simulink library "UpmixerLib"  (R2022b)
settings: Solver=VariableStepAuto  StartTime=0.0  StopTime=10.0  RelTol=1e-3
undefined symbols (not defined in the file or in its folder): carModel, mode, upmixer
libraries: TuneVar x40, MixerLib x31, $bdroot x13, FeaturePath x6, RTC x4
settings Model: Creator=ak1044356  LastModifiedBy=sa1045272
settings SolverCC: AlgebraicLoopSolver=TrustRegion
settings DebuggingCC: UnconnectedInputMsg=warning  UnconnectedOutputMsg=warning  UnconnectedLineMsg=warning  SFMachineParentedDataDiag=warning  ArithmeticOperatorsInVariantConditions=warning
settings ModelReferenceCC: EnableRefExpFcnMdlSchedulingChecks=on
settings SFSimCC: CustomCodeUndefinedFunction=UseInterfaceOnly

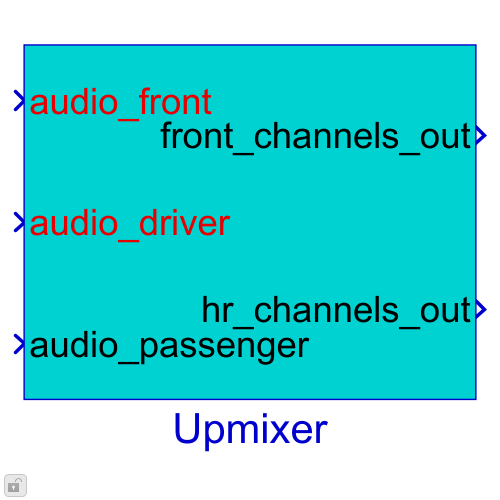
[thumbnail: Simulink's stored preview of the top-level diagram]
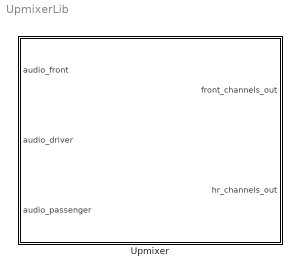
== system UpmixerLib ==
  Upmixer : Subsystem  InitFcn=|
      | upmixer.front_peripheral_channel_count = min(upmixer.front_peripheral_channel_count, 7);
      | upmixer.front_peripheral_channel_count = max(upmixer.front_peripheral_channel_count, 2);
      | upmixer.headrest_count = min(upmixer.headrest_count, 2);
      | upmixer.headrest_count = max(upmixer.headrest_count, 1);

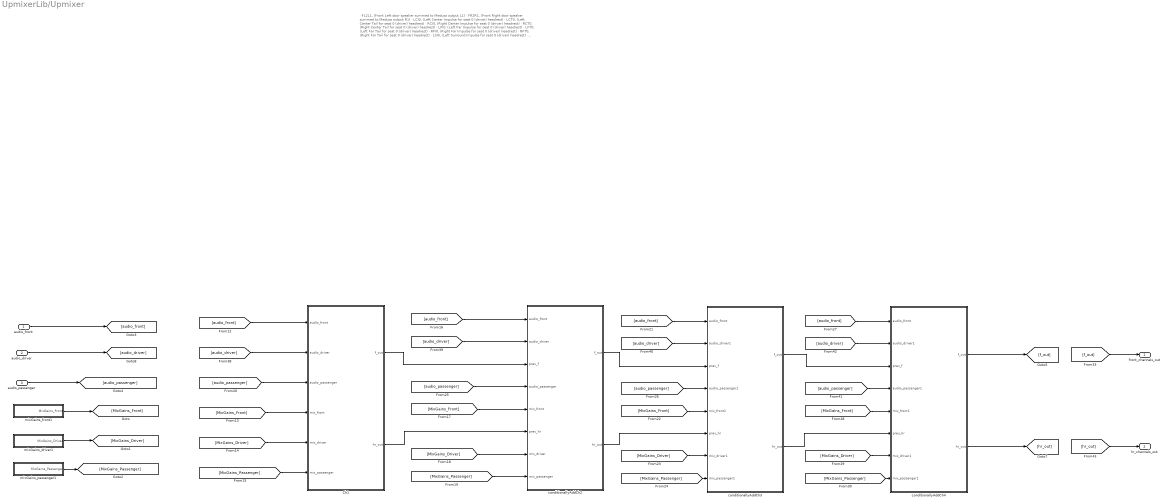
== system UpmixerLib/Upmixer ==
  note: · FL2L1, (Front Left door speaker summed to Medusa output L1)
      | · FR2R1, (Front Right door speaker summed to Medusa output R1)
      | · LCI0, (Left Center Impulse for seat 0 (driver) headrest)
      | · LCT0, (Left Center Tail for seat 0 (driver) headrest)
      | · RCI0, (Right Center Impulse for seat 0 (driver) headrest)
      | · RCT0, (Right Center Tail for seat 0 (driver) headrest)
      | · LFI0, (Left Far Impulse for seat 0 (driver) headrest)
      | · LFT0, (Left Far Tail for seat 0 (driver) headrest)
      | · RFI0, (Right Far Impulse for seat 0 (driver) headrest)
      | · RFT0, (Right Far Tail for seat 0 (driver) headrest)
      | · LSI0, (Left Surround Impulse for seat 0 (driver) headrest)
      | · LST0, (Left Surround Tail for seat 0 (driver) headrest)
      | · RSI0, (Right Surround Impulse for seat 0 (driver) headrest)
      | · RST0 (Right Surround Tail for seat 0 (driver) headrest)
  audio_front : Inport
  audio_driver : Inport  Port=2
  audio_passenger : Inport  Port=3
  Ch1 : Subsystem
  conditionallyAddCh2 : Subsystem
  conditionallyAddCh3 : Subsystem  AncestorBlock=UpmixerLib/Upmixer/conditionallyAddCh2
      settings: LibrarySourceBlock=UpmixerLib/Upmixer/conditionallyAddCh2
  conditionallyAddCh4 : Subsystem  AncestorBlock=UpmixerLib/Upmixer/conditionallyAddCh2
      settings: LibrarySourceBlock=UpmixerLib/Upmixer/conditionallyAddCh2
  mixGains_driver1 : Subsystem
  mixGains_front1 : Subsystem
  mixGains_passenger1 : Subsystem
  front_channels_out : Outport  VectorParamsAs1DForOutWhenUnconnected=off
  hr_channels_out : Outport  Port=2  VectorParamsAs1DForOutWhenUnconnected=off
  wires:
  mixGains_front1/1(MixGains_Front) -> [MixGains_Front]
  mixGains_driver1/1(MixGains_Driver) -> [MixGains_Driver]
  mixGains_passenger1/1(MixGains_Passenger) -> [MixGains_Passenger]
  audio_front/1 -> [audio_front]
  [audio_front] -> conditionallyAddCh2/1(audio_front)
  [MixGains_Front] -> conditionallyAddCh2/5(mix_front)
  [MixGains_Driver] -> conditionallyAddCh2/7(mix_driver)
  [MixGains_Passenger] -> conditionallyAddCh2/8(mix_passenger)
  [f_out] -> front_channels_out/1
  audio_driver/1 -> [audio_driver]
  [audio_driver] -> conditionallyAddCh2/2(audio_driver)
  [audio_front] -> Ch1/1(audio_front)
  [audio_driver] -> Ch1/2(audio_driver)
  [MixGains_Front] -> Ch1/4(mix_front)
  [MixGains_Driver] -> Ch1/5(mix_driver)
  [MixGains_Passenger] -> Ch1/6(mix_passenger)
  conditionallyAddCh4/1(f_out) -> [f_out]
  audio_passenger/1 -> [audio_passenger]
  [audio_passenger] -> Ch1/3(audio_passenger)
  [audio_passenger] -> conditionallyAddCh2/4(audio_passenger)
  Ch1/1(f_out) -> conditionallyAddCh2/3(prev_f)
  Ch1/2(hr_out) -> conditionallyAddCh2/6(prev_hr)
  [MixGains_Front] -> conditionallyAddCh3/5(mix_front1)
  [audio_front] -> conditionallyAddCh3/1(audio_front)
  [MixGains_Passenger] -> conditionallyAddCh3/8(mix_passenger1)
  [audio_driver] -> conditionallyAddCh3/2(audio_driver1)
  [audio_passenger] -> conditionallyAddCh3/4(audio_passenger1)
  [MixGains_Driver] -> conditionallyAddCh3/7(mix_driver1)
  conditionallyAddCh2/2(hr_out) -> conditionallyAddCh3/6(prev_hr)
  conditionallyAddCh2/1(f_out) -> conditionallyAddCh3/3(prev_f)
  conditionallyAddCh3/1(f_out) -> conditionallyAddCh4/3(prev_f)
  conditionallyAddCh3/2(hr_out) -> conditionallyAddCh4/6(prev_hr)
  [audio_front] -> conditionallyAddCh4/1(audio_front)
  [audio_driver] -> conditionallyAddCh4/2(audio_driver1)
  [audio_passenger] -> conditionallyAddCh4/4(audio_passenger1)
  [MixGains_Front] -> conditionallyAddCh4/5(mix_front1)
  [MixGains_Driver] -> conditionallyAddCh4/7(mix_driver1)
  [MixGains_Passenger] -> conditionallyAddCh4/8(mix_passenger1)
  conditionallyAddCh4/2(hr_out) -> [hr_out]
  [hr_out] -> hr_channels_out/1

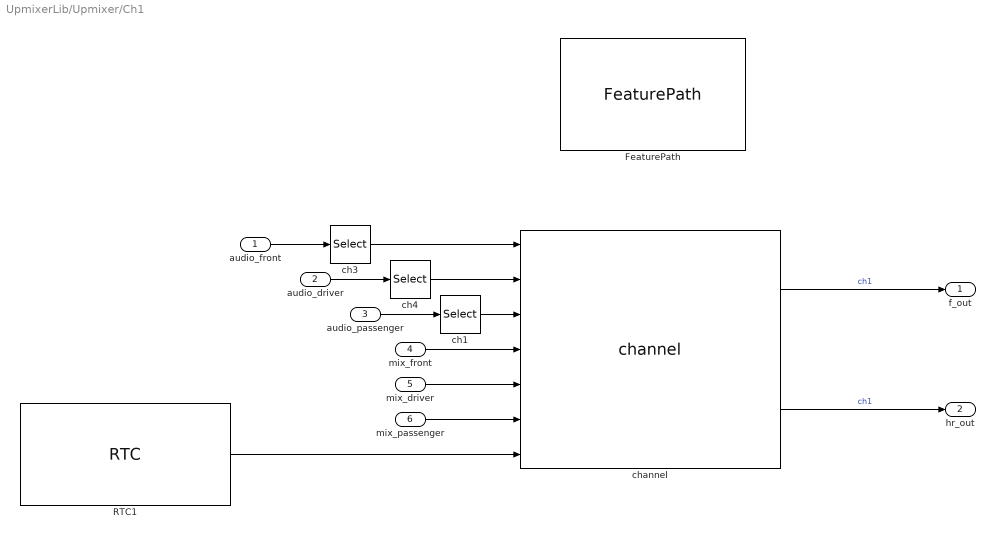
== system UpmixerLib/Upmixer/Ch1 ==
  audio_front : Inport
  audio_driver : Inport  Port=2
  audio_passenger : Inport  Port=3
  mix_front : Inport  Port=4
  mix_driver : Inport  Port=5
  mix_passenger : Inport  Port=6
  FeaturePath : FeaturePath/FeaturePath  FeatureName=Channel1_  IsGroup=off  GroupNumber=-1  DeclarePackages=off  PackageNames=mode,carModel  IsToolGroup=off  TriggerInit=[310 -171 495 -59]
  RTC1 : RTC/RTC  REQ_Priority=RTC_Mask.NormalPriority  RequestAtInit=off  EnableRequest=off  REQElemName1=loc  REQElemType1=single  REQElemWidth1=2  REQElemInitial1=upmixer.loc_init  REQElemType2=uint32  REQElemWidth2=1  REQElemInitial2=[]  REQElemType3=uint32  REQElemWidth3=1  REQElemInitial3=[]  REQElemType4=uint32  REQElemWidth4=1  REQElemInitial4=[]  REQElemType5=uint32  REQElemWidth5=1  REQElemInitial5=[]  REQElemType6=uint32  REQElemWidth6=1  REQElemInitial6=[]  REQElemType7=uint32  REQElemWidth7=1  REQElemInitial7=[]  REQElemType8=uint32  REQElemWidth8=1  REQElemInitial8=[]  REQElemType9=uint32  REQElemWidth9=1  REQElemInitial9=[]  REQElemType10=uint32  REQElemWidth10=1  REQElemInitial10=[]  EnableResponse=on  EnableRSP_StatusIn=off  RSPElemType1=single  RSPElemWidth1=1  RSPElemType2=uint32  RSPElemWidth2=1  RSPElemType3=uint32  RSPElemWidth3=1  RSPElemType4=uint32  RSPElemWidth4=1  RSPElemType5=uint32  RSPElemWidth5=1  RSPElemType6=uint32  RSPElemWidth6=1  RSPElemType7=uint32  RSPElemWidth7=1  RSPElemType8=uint32  RSPElemWidth8=1  RSPElemType9=uint32  RSPElemWidth9=1  RSPElemType10=uint32  RSPElemWidth10=1  EnableNotification=off  EnableNTF_PrepTrig=off  NTFElemType1=uint32  NTFElemWidth1=1  NTFElemType2=uint32  NTFElemWidth2=1  NTFElemType3=uint32  NTFElemWidth3=1  NTFElemType4=uint32  NTFElemWidth4=1  NTFElemType5=uint32  NTFElemWidth5=1  NTFElemType6=uint32  NTFElemWidth6=1  NTFElemType7=uint32  NTFElemWidth7=1  NTFElemType8=uint32  NTFElemWidth8=1  NTFElemType9=uint32  NTFElemWidth9=1  NTFElemType10=uint32  NTFElemWidth10=1  MaskMessageName=Location
  ch1 : Selector  NumberOfDimensions=2  InputPortWidth=3  IndexOptions=Select all,Index vector (dialog)  Indices=4,min(1, upmixer.ann_sysin_channel_count)  OutputSizes=1,1
  ch3 : Selector  NumberOfDimensions=2  InputPortWidth=3  IndexOptions=Select all,Index vector (dialog)  Indices=4,min(1, upmixer.ann_sysin_channel_count)  OutputSizes=1,1
  ch4 : Selector  NumberOfDimensions=2  InputPortWidth=3  IndexOptions=Select all,Index vector (dialog)  Indices=4,min(1, upmixer.ann_sysin_channel_count)  OutputSizes=1,1
  channel : $bdroot/Upmixer/conditionallyAddCh2/If Action Subsystem1/channel  SystemSampleTime=-1  VariantActivationTime=update diagram  Latency=0  AutoFrameSizeCalculation=off
  f_out : Outport  VectorParamsAs1DForOutWhenUnconnected=off
  hr_out : Outport  Port=2  VectorParamsAs1DForOutWhenUnconnected=off
  wires:
  mix_front/1 -> channel/4
  audio_front/1 -> ch3/1
  mix_driver/1 -> channel/5
  mix_passenger/1 -> channel/6
  channel/1 -> f_out/1  "ch1"
  audio_driver/1 -> ch4/1
  RTC1/1 -> channel/7
  audio_passenger/1 -> ch1/1
  ch1/1 -> channel/3
  ch4/1 -> channel/2
  ch3/1 -> channel/1
  channel/2 -> hr_out/1  "ch1"

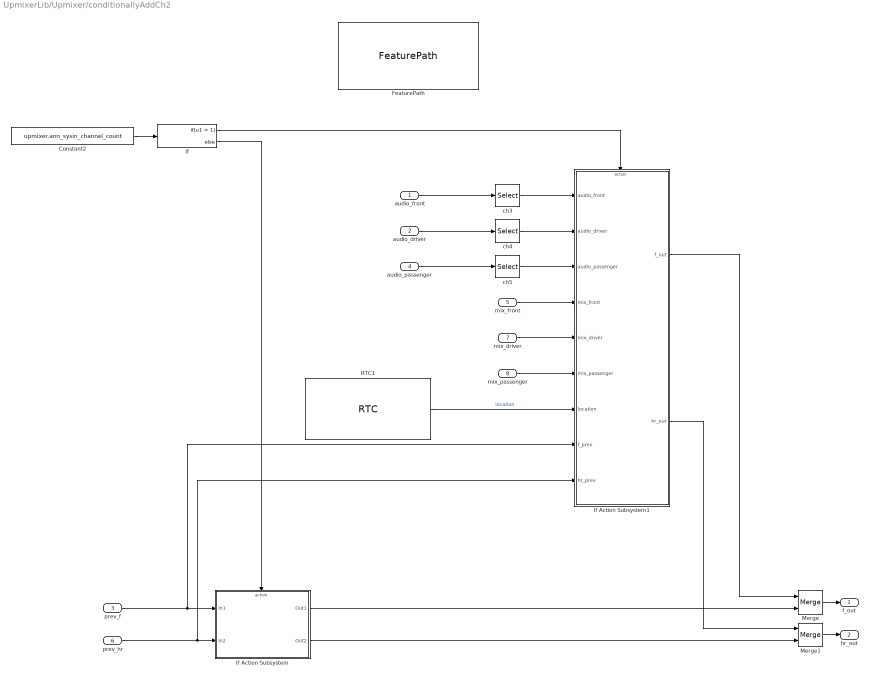
== system UpmixerLib/Upmixer/conditionallyAddCh2 ==
  audio_front : Inport
  audio_driver : Inport  Port=2
  prev_f : Inport  Port=3
  audio_passenger : Inport  Port=4
  mix_front : Inport  Port=5
  prev_hr : Inport  Port=6
  mix_driver : Inport  Port=7
  mix_passenger : Inport  Port=8
  Constant2 : Constant  Value=upmixer.ann_sysin_channel_count
  FeaturePath : FeaturePath/FeaturePath  FeatureName=Channel2_  IsGroup=off  GroupNumber=-1  DeclarePackages=off  PackageNames=mode,carModel  IsToolGroup=off  TriggerInit=[515 -436 750 -324]
  If : If  IfExpression=u1 > 1
  If Action Subsystem : Subsystem  TreatAsAtomicUnit=on
  If Action Subsystem1 : Subsystem  TreatAsAtomicUnit=on
  Merge : Merge
  Merge1 : Merge
  RTC1 : RTC/RTC  REQ_Priority=RTC_Mask.NormalPriority  RequestAtInit=off  EnableRequest=off  REQElemName1=loc  REQElemType1=single  REQElemWidth1=2  REQElemInitial1=upmixer.loc_init  REQElemType2=uint32  REQElemWidth2=1  REQElemInitial2=[]  REQElemType3=uint32  REQElemWidth3=1  REQElemInitial3=[]  REQElemType4=uint32  REQElemWidth4=1  REQElemInitial4=[]  REQElemType5=uint32  REQElemWidth5=1  REQElemInitial5=[]  REQElemType6=uint32  REQElemWidth6=1  REQElemInitial6=[]  REQElemType7=uint32  REQElemWidth7=1  REQElemInitial7=[]  REQElemType8=uint32  REQElemWidth8=1  REQElemInitial8=[]  REQElemType9=uint32  REQElemWidth9=1  REQElemInitial9=[]  REQElemType10=uint32  REQElemWidth10=1  REQElemInitial10=[]  EnableResponse=on  EnableRSP_StatusIn=off  RSPElemType1=single  RSPElemWidth1=1  RSPElemType2=uint32  RSPElemWidth2=1  RSPElemType3=uint32  RSPElemWidth3=1  RSPElemType4=uint32  RSPElemWidth4=1  RSPElemType5=uint32  RSPElemWidth5=1  RSPElemType6=uint32  RSPElemWidth6=1  RSPElemType7=uint32  RSPElemWidth7=1  RSPElemType8=uint32  RSPElemWidth8=1  RSPElemType9=uint32  RSPElemWidth9=1  RSPElemType10=uint32  RSPElemWidth10=1  EnableNotification=off  EnableNTF_PrepTrig=off  NTFElemType1=uint32  NTFElemWidth1=1  NTFElemType2=uint32  NTFElemWidth2=1  NTFElemType3=uint32  NTFElemWidth3=1  NTFElemType4=uint32  NTFElemWidth4=1  NTFElemType5=uint32  NTFElemWidth5=1  NTFElemType6=uint32  NTFElemWidth6=1  NTFElemType7=uint32  NTFElemWidth7=1  NTFElemType8=uint32  NTFElemWidth8=1  NTFElemType9=uint32  NTFElemWidth9=1  NTFElemType10=uint32  NTFElemWidth10=1  MaskMessageName=Location
  ch3 : Selector  NumberOfDimensions=2  InputPortWidth=3  IndexOptions=Select all,Index vector (dialog)  Indices=4,min(2, upmixer.ann_sysin_channel_count)  OutputSizes=1,1
  ch4 : Selector  NumberOfDimensions=2  InputPortWidth=3  IndexOptions=Select all,Index vector (dialog)  Indices=4,min(2, upmixer.ann_sysin_channel_count)  OutputSizes=1,1
  ch5 : Selector  NumberOfDimensions=2  InputPortWidth=3  IndexOptions=Select all,Index vector (dialog)  Indices=4,min(2, upmixer.ann_sysin_channel_count)  OutputSizes=1,1
  f_out : Outport  VectorParamsAs1DForOutWhenUnconnected=off
  hr_out : Outport  Port=2  VectorParamsAs1DForOutWhenUnconnected=off
  wires:
  Constant2/1 -> If/1
  If/2 -> If Action Subsystem/Action
  prev_f/1 -> If Action Subsystem1/8(f_prev), If Action Subsystem/1(In1)
  If/1 -> If Action Subsystem1/Action
  audio_front/1 -> ch3/1
  If Action Subsystem/1(Out1) -> Merge/2
  If Action Subsystem1/1(f_out) -> Merge/1
  Merge/1 -> f_out/1
  mix_front/1 -> If Action Subsystem1/4(mix_front)
  mix_driver/1 -> If Action Subsystem1/5(mix_driver)
  mix_passenger/1 -> If Action Subsystem1/6(mix_passenger)
  RTC1/1 -> If Action Subsystem1/7(location)  "location"
  ch3/1 -> If Action Subsystem1/1(audio_front)
  audio_driver/1 -> ch4/1
  ch4/1 -> If Action Subsystem1/2(audio_driver)
  audio_passenger/1 -> ch5/1
  ch5/1 -> If Action Subsystem1/3(audio_passenger)
  prev_hr/1 -> If Action Subsystem1/9(hr_prev), If Action Subsystem/2(In2)
  If Action Subsystem/2(Out2) -> Merge1/2
  If Action Subsystem1/2(hr_out) -> Merge1/1
  Merge1/1 -> hr_out/1

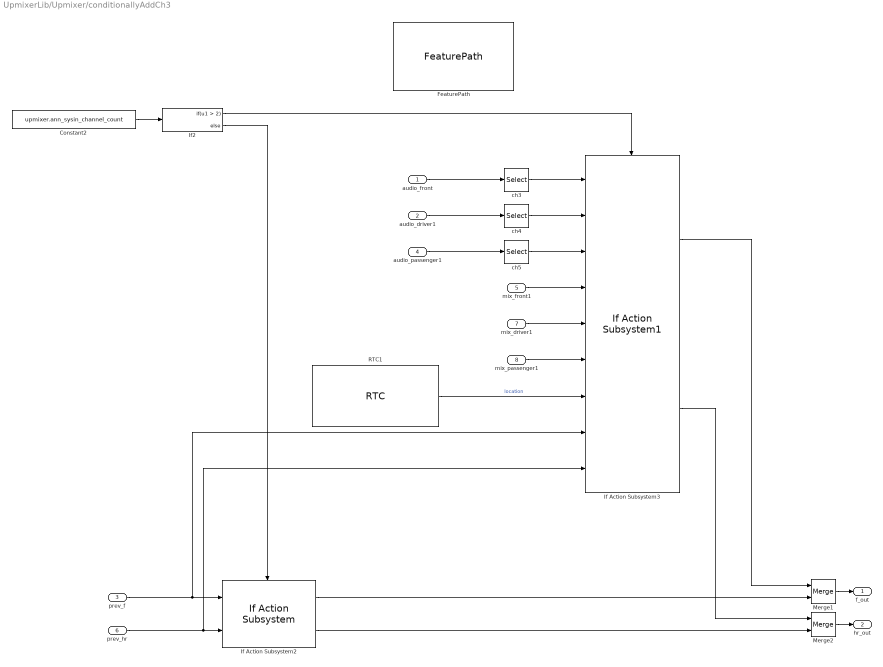
== system UpmixerLib/Upmixer/conditionallyAddCh3 ==
  audio_front : Inport
  audio_driver1 : Inport  Port=2
  prev_f : Inport  Port=3
  audio_passenger1 : Inport  Port=4
  mix_front1 : Inport  Port=5
  prev_hr : Inport  Port=6
  mix_driver1 : Inport  Port=7
  mix_passenger1 : Inport  Port=8
  Constant2 : Constant  Value=upmixer.ann_sysin_channel_count
  FeaturePath : FeaturePath/FeaturePath  FeatureName=Channel3_  IsGroup=off  GroupNumber=-1  DeclarePackages=off  PackageNames=mode,carModel  IsToolGroup=off  TriggerInit=[860 2299 1060 2411]
  If Action Subsystem2 : $bdroot/Upmixer/conditionallyAddCh2/If Action Subsystem  SystemSampleTime=-1  VariantActivationTime=update diagram  Latency=0  AutoFrameSizeCalculation=off
  If Action Subsystem3 : $bdroot/Upmixer/conditionallyAddCh2/If Action Subsystem1  SystemSampleTime=-1  VariantActivationTime=update diagram  Latency=0  AutoFrameSizeCalculation=off
  If2 : If  IfExpression=u1 > 2
  Merge1 : Merge
  Merge2 : Merge
  RTC1 : RTC/RTC  REQ_Priority=RTC_Mask.NormalPriority  RequestAtInit=off  EnableRequest=off  REQElemName1=loc  REQElemType1=single  REQElemWidth1=2  REQElemInitial1=upmixer.loc_init  REQElemType2=uint32  REQElemWidth2=1  REQElemInitial2=[]  REQElemType3=uint32  REQElemWidth3=1  REQElemInitial3=[]  REQElemType4=uint32  REQElemWidth4=1  REQElemInitial4=[]  REQElemType5=uint32  REQElemWidth5=1  REQElemInitial5=[]  REQElemType6=uint32  REQElemWidth6=1  REQElemInitial6=[]  REQElemType7=uint32  REQElemWidth7=1  REQElemInitial7=[]  REQElemType8=uint32  REQElemWidth8=1  REQElemInitial8=[]  REQElemType9=uint32  REQElemWidth9=1  REQElemInitial9=[]  REQElemType10=uint32  REQElemWidth10=1  REQElemInitial10=[]  EnableResponse=on  EnableRSP_StatusIn=off  RSPElemType1=single  RSPElemWidth1=1  RSPElemType2=uint32  RSPElemWidth2=1  RSPElemType3=uint32  RSPElemWidth3=1  RSPElemType4=uint32  RSPElemWidth4=1  RSPElemType5=uint32  RSPElemWidth5=1  RSPElemType6=uint32  RSPElemWidth6=1  RSPElemType7=uint32  RSPElemWidth7=1  RSPElemType8=uint32  RSPElemWidth8=1  RSPElemType9=uint32  RSPElemWidth9=1  RSPElemType10=uint32  RSPElemWidth10=1  EnableNotification=off  EnableNTF_PrepTrig=off  NTFElemType1=uint32  NTFElemWidth1=1  NTFElemType2=uint32  NTFElemWidth2=1  NTFElemType3=uint32  NTFElemWidth3=1  NTFElemType4=uint32  NTFElemWidth4=1  NTFElemType5=uint32  NTFElemWidth5=1  NTFElemType6=uint32  NTFElemWidth6=1  NTFElemType7=uint32  NTFElemWidth7=1  NTFElemType8=uint32  NTFElemWidth8=1  NTFElemType9=uint32  NTFElemWidth9=1  NTFElemType10=uint32  NTFElemWidth10=1  MaskMessageName=Location
  ch3 : Selector  NumberOfDimensions=2  InputPortWidth=3  IndexOptions=Select all,Index vector (dialog)  Indices=4,min(3, upmixer.ann_sysin_channel_count)  OutputSizes=1,1
  ch4 : Selector  NumberOfDimensions=2  InputPortWidth=3  IndexOptions=Select all,Index vector (dialog)  Indices=4,min(3, upmixer.ann_sysin_channel_count)  OutputSizes=1,1
  ch5 : Selector  NumberOfDimensions=2  InputPortWidth=3  IndexOptions=Select all,Index vector (dialog)  Indices=4,min(3, upmixer.ann_sysin_channel_count)  OutputSizes=1,1
  f_out : Outport  VectorParamsAs1DForOutWhenUnconnected=off
  hr_out : Outport  Port=2  VectorParamsAs1DForOutWhenUnconnected=off
  wires:
  If Action Subsystem2/2 -> Merge2/2
  prev_hr/1 -> If Action Subsystem3/9, If Action Subsystem2/2
  ch4/1 -> If Action Subsystem3/2
  If Action Subsystem2/1 -> Merge1/2
  ch5/1 -> If Action Subsystem3/3
  Merge1/1 -> f_out/1
  audio_passenger1/1 -> ch5/1
  audio_driver1/1 -> ch4/1
  prev_f/1 -> If Action Subsystem3/8, If Action Subsystem2/1
  audio_front/1 -> ch3/1
  mix_passenger1/1 -> If Action Subsystem3/6
  If Action Subsystem3/1 -> Merge1/1
  If Action Subsystem3/2 -> Merge2/1
  RTC1/1 -> If Action Subsystem3/7  "location"
  mix_driver1/1 -> If Action Subsystem3/5
  If2/1 -> If Action Subsystem3/Action
  If2/2 -> If Action Subsystem2/Action
  mix_front1/1 -> If Action Subsystem3/4
  ch3/1 -> If Action Subsystem3/1
  Constant2/1 -> If2/1
  Merge2/1 -> hr_out/1

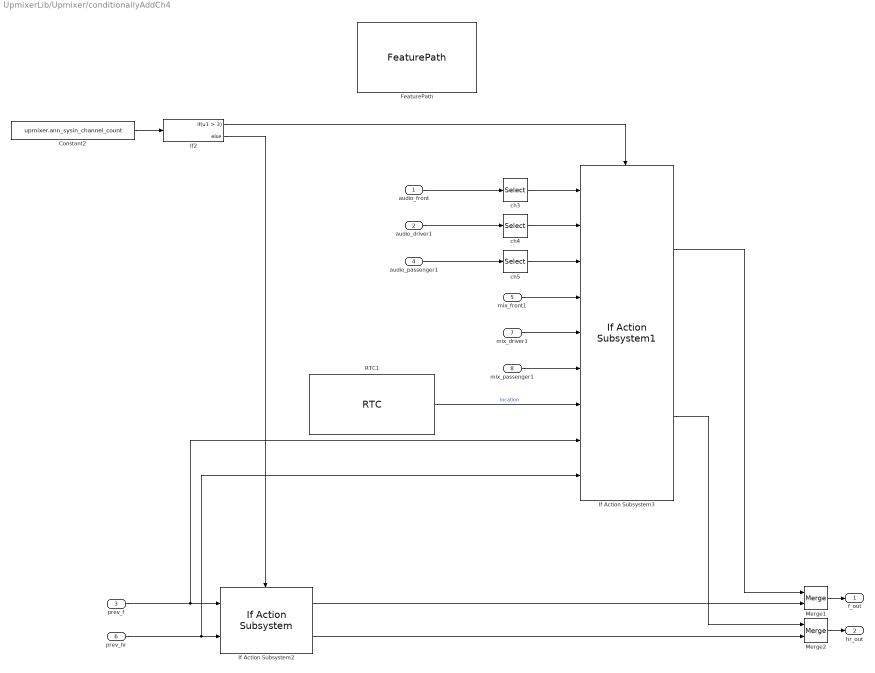
== system UpmixerLib/Upmixer/conditionallyAddCh4 ==
  audio_front : Inport
  audio_driver1 : Inport  Port=2
  prev_f : Inport  Port=3
  audio_passenger1 : Inport  Port=4
  mix_front1 : Inport  Port=5
  prev_hr : Inport  Port=6
  mix_driver1 : Inport  Port=7
  mix_passenger1 : Inport  Port=8
  Constant2 : Constant  Value=upmixer.ann_sysin_channel_count
  FeaturePath : FeaturePath/FeaturePath  FeatureName=Channel4_  IsGroup=off  GroupNumber=-1  DeclarePackages=off  PackageNames=mode,carModel  IsToolGroup=off  TriggerInit=[750 2239 950 2356]
  If Action Subsystem2 : $bdroot/Upmixer/conditionallyAddCh2/If Action Subsystem  SystemSampleTime=-1  VariantActivationTime=update diagram  Latency=0  AutoFrameSizeCalculation=off
  If Action Subsystem3 : $bdroot/Upmixer/conditionallyAddCh2/If Action Subsystem1  SystemSampleTime=-1  VariantActivationTime=update diagram  Latency=0  AutoFrameSizeCalculation=off
  If2 : If  IfExpression=u1 > 3
  Merge1 : Merge
  Merge2 : Merge
  RTC1 : RTC/RTC  REQ_Priority=RTC_Mask.NormalPriority  RequestAtInit=off  EnableRequest=off  REQElemName1=loc  REQElemType1=single  REQElemWidth1=2  REQElemInitial1=upmixer.loc_init  REQElemType2=uint32  REQElemWidth2=1  REQElemInitial2=[]  REQElemType3=uint32  REQElemWidth3=1  REQElemInitial3=[]  REQElemType4=uint32  REQElemWidth4=1  REQElemInitial4=[]  REQElemType5=uint32  REQElemWidth5=1  REQElemInitial5=[]  REQElemType6=uint32  REQElemWidth6=1  REQElemInitial6=[]  REQElemType7=uint32  REQElemWidth7=1  REQElemInitial7=[]  REQElemType8=uint32  REQElemWidth8=1  REQElemInitial8=[]  REQElemType9=uint32  REQElemWidth9=1  REQElemInitial9=[]  REQElemType10=uint32  REQElemWidth10=1  REQElemInitial10=[]  EnableResponse=on  EnableRSP_StatusIn=off  RSPElemType1=single  RSPElemWidth1=1  RSPElemType2=uint32  RSPElemWidth2=1  RSPElemType3=uint32  RSPElemWidth3=1  RSPElemType4=uint32  RSPElemWidth4=1  RSPElemType5=uint32  RSPElemWidth5=1  RSPElemType6=uint32  RSPElemWidth6=1  RSPElemType7=uint32  RSPElemWidth7=1  RSPElemType8=uint32  RSPElemWidth8=1  RSPElemType9=uint32  RSPElemWidth9=1  RSPElemType10=uint32  RSPElemWidth10=1  EnableNotification=off  EnableNTF_PrepTrig=off  NTFElemType1=uint32  NTFElemWidth1=1  NTFElemType2=uint32  NTFElemWidth2=1  NTFElemType3=uint32  NTFElemWidth3=1  NTFElemType4=uint32  NTFElemWidth4=1  NTFElemType5=uint32  NTFElemWidth5=1  NTFElemType6=uint32  NTFElemWidth6=1  NTFElemType7=uint32  NTFElemWidth7=1  NTFElemType8=uint32  NTFElemWidth8=1  NTFElemType9=uint32  NTFElemWidth9=1  NTFElemType10=uint32  NTFElemWidth10=1  MaskMessageName=Location
  ch3 : Selector  NumberOfDimensions=2  InputPortWidth=3  IndexOptions=Select all,Index vector (dialog)  Indices=4,min(4, upmixer.ann_sysin_channel_count)  OutputSizes=1,1
  ch4 : Selector  NumberOfDimensions=2  InputPortWidth=3  IndexOptions=Select all,Index vector (dialog)  Indices=4,min(4, upmixer.ann_sysin_channel_count)  OutputSizes=1,1
  ch5 : Selector  NumberOfDimensions=2  InputPortWidth=3  IndexOptions=Select all,Index vector (dialog)  Indices=4,min(4, upmixer.ann_sysin_channel_count)  OutputSizes=1,1
  f_out : Outport  VectorParamsAs1DForOutWhenUnconnected=off
  hr_out : Outport  Port=2  VectorParamsAs1DForOutWhenUnconnected=off
  wires:
  If2/1 -> If Action Subsystem3/Action
  Constant2/1 -> If2/1
  ch4/1 -> If Action Subsystem3/2
  audio_driver1/1 -> ch4/1
  If2/2 -> If Action Subsystem2/Action
  RTC1/1 -> If Action Subsystem3/7  "location"
  Merge2/1 -> hr_out/1
  mix_driver1/1 -> If Action Subsystem3/5
  If Action Subsystem3/2 -> Merge2/1
  mix_front1/1 -> If Action Subsystem3/4
  Merge1/1 -> f_out/1
  prev_f/1 -> If Action Subsystem3/8, If Action Subsystem2/1
  mix_passenger1/1 -> If Action Subsystem3/6
  prev_hr/1 -> If Action Subsystem3/9, If Action Subsystem2/2
  If Action Subsystem2/2 -> Merge2/2
  audio_front/1 -> ch3/1
  If Action Subsystem2/1 -> Merge1/2
  If Action Subsystem3/1 -> Merge1/1
  audio_passenger1/1 -> ch5/1
  ch3/1 -> If Action Subsystem3/1
  ch5/1 -> If Action Subsystem3/3

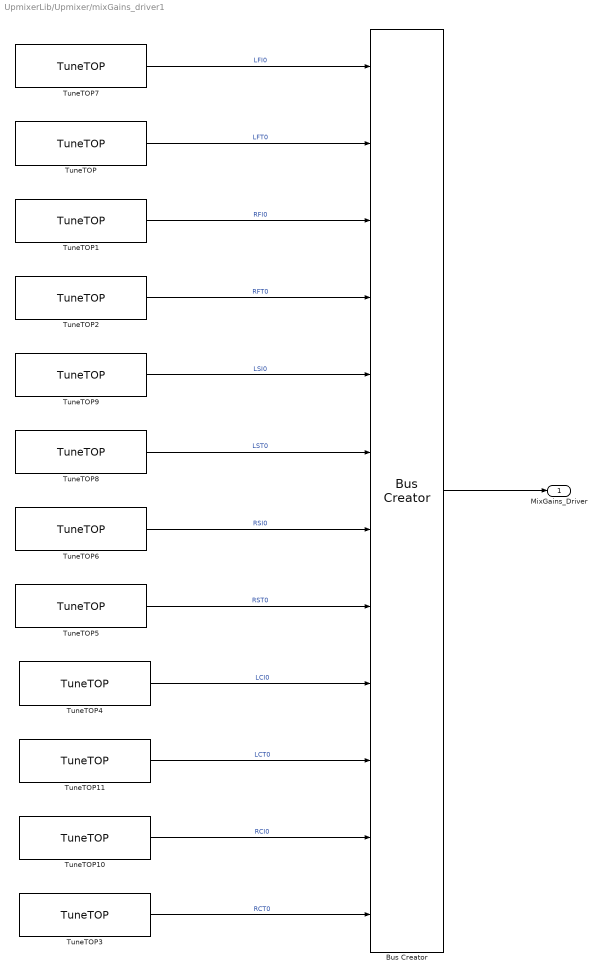
== system UpmixerLib/Upmixer/mixGains_driver1 ==
  Bus Creator : BusCreator  Inputs=12
  TuneTOP : TuneVar/TuneTOP  TriggerInit=[4795 907 4965 963]  TopName=LFT0_mix  TuneName=LFT0_mix  DataType=single  PackageName=mode  BankNumber=0  TunabilityNumber=1  MinValue=[]  MaxValue=[]  UseSameName=on  MaskValue=upmixer.mix.LFT0
  TuneTOP1 : TuneVar/TuneTOP  TriggerInit=[4795 1007 4965 1063]  TopName=RFI0_mix  TuneName=RFI0_mix  DataType=single  PackageName=mode  BankNumber=0  TunabilityNumber=1  MinValue=[]  MaxValue=[]  UseSameName=on  MaskValue=upmixer.mix.RFI0
  TuneTOP10 : TuneVar/TuneTOP  TriggerInit=[4800 1807 4970 1863]  TopName=RCI0_mix  TuneName=RCI0_mix  DataType=single  PackageName=mode  BankNumber=0  TunabilityNumber=1  MinValue=[]  MaxValue=[]  UseSameName=on  MaskValue=upmixer.mix.RCI0
  TuneTOP11 : TuneVar/TuneTOP  TriggerInit=[4800 1707 4970 1763]  TopName=LCT0_mix  TuneName=LCT0_mix  DataType=single  PackageName=mode  BankNumber=0  TunabilityNumber=1  MinValue=[]  MaxValue=[]  UseSameName=on  MaskValue=upmixer.mix.LCT0
  TuneTOP2 : TuneVar/TuneTOP  TriggerInit=[4795 1107 4965 1163]  TopName=RFT0_mix  TuneName=RFT0_mix  DataType=single  PackageName=mode  BankNumber=0  TunabilityNumber=1  MinValue=[]  MaxValue=[]  UseSameName=on  MaskValue=upmixer.mix.RFT0
  TuneTOP3 : TuneVar/TuneTOP  TriggerInit=[4800 1907 4970 1963]  TopName=RCT0_mix  TuneName=RCT0_mix  DataType=single  PackageName=mode  BankNumber=0  TunabilityNumber=1  MinValue=[]  MaxValue=[]  UseSameName=on  MaskValue=upmixer.mix.RCT0
  TuneTOP4 : TuneVar/TuneTOP  TriggerInit=[4800 1607 4970 1663]  TopName=LCI0_mix  TuneName=LCI0_mix  DataType=single  PackageName=mode  BankNumber=0  TunabilityNumber=1  MinValue=[]  MaxValue=[]  UseSameName=on  MaskValue=upmixer.mix.LCI0
  TuneTOP5 : TuneVar/TuneTOP  TriggerInit=[4795 1507 4965 1563]  TopName=RST0_mix  TuneName=RST0_mix  DataType=single  PackageName=mode  BankNumber=0  TunabilityNumber=1  MinValue=[]  MaxValue=[]  UseSameName=on  MaskValue=upmixer.mix.RST0
  TuneTOP6 : TuneVar/TuneTOP  TriggerInit=[4795 1407 4965 1463]  TopName=RSI0_mix  TuneName=RSI0_mix  DataType=single  PackageName=mode  BankNumber=0  TunabilityNumber=1  MinValue=[]  MaxValue=[]  UseSameName=on  MaskValue=upmixer.mix.RSI0
  TuneTOP7 : TuneVar/TuneTOP  TriggerInit=[4795 807 4965 863]  TopName=LFI0_mix  TuneName=LFI0_mix  DataType=single  PackageName=mode  BankNumber=0  TunabilityNumber=1  MinValue=[]  MaxValue=[]  UseSameName=on  MaskValue=upmixer.mix.LFI0
  TuneTOP8 : TuneVar/TuneTOP  TriggerInit=[4795 1307 4965 1363]  TopName=LST0_mix  TuneName=LST0_mix  DataType=single  PackageName=mode  BankNumber=0  TunabilityNumber=1  MinValue=[]  MaxValue=[]  UseSameName=on  MaskValue=upmixer.mix.LST0
  TuneTOP9 : TuneVar/TuneTOP  TriggerInit=[4795 1207 4965 1263]  TopName=LSI0_mix  TuneName=LSI0_mix  DataType=single  PackageName=mode  BankNumber=0  TunabilityNumber=1  MinValue=[]  MaxValue=[]  UseSameName=on  MaskValue=upmixer.mix.LSI0
  MixGains_Driver : Outport  VectorParamsAs1DForOutWhenUnconnected=off
  wires:
  TuneTOP7/1 -> Bus Creator/1  "LFI0"
  TuneTOP/1 -> Bus Creator/2  "LFT0"
  TuneTOP1/1 -> Bus Creator/3  "RFI0"
  TuneTOP2/1 -> Bus Creator/4  "RFT0"
  TuneTOP9/1 -> Bus Creator/5  "LSI0"
  TuneTOP8/1 -> Bus Creator/6  "LST0"
  TuneTOP6/1 -> Bus Creator/7  "RSI0"
  TuneTOP5/1 -> Bus Creator/8  "RST0"
  TuneTOP4/1 -> Bus Creator/9  "LCI0"
  TuneTOP11/1 -> Bus Creator/10  "LCT0"
  TuneTOP10/1 -> Bus Creator/11  "RCI0"
  TuneTOP3/1 -> Bus Creator/12  "RCT0"
  Bus Creator/1 -> MixGains_Driver/1

== system UpmixerLib/Upmixer/mixGains_front1 ==
  Bus Creator : BusCreator  Inputs=7
  TuneTOP : TuneVar/TuneTOP  TriggerInit=[1050 32 1220 88]  TopName=dc_mix  TuneName=dc_mix  DataType=single  PackageName=mode  BankNumber=0  TunabilityNumber=1  MinValue=[]  MaxValue=[]  UseSameName=on  MaskValue=upmixer.mix.dc
  TuneTOP1 : TuneVar/TuneTOP  TriggerInit=[1050 167 1220 223]  TopName=fl_mix  TuneName=fl_mix  DataType=single  PackageName=mode  BankNumber=0  TunabilityNumber=1  MinValue=[]  MaxValue=[]  UseSameName=on  MaskValue=upmixer.mix.fl
  TuneTOP2 : TuneVar/TuneTOP  TriggerInit=[1050 302 1220 358]  TopName=fr_mix  TuneName=fr_mix  DataType=single  PackageName=mode  BankNumber=0  TunabilityNumber=1  MinValue=[]  MaxValue=[]  UseSameName=on  MaskValue=upmixer.mix.fr
  TuneTOP3 : TuneVar/TuneTOP  TriggerInit=[1050 842 1220 898]  TopName=frw_mix  TuneName=frw_mix  DataType=single  PackageName=mode  BankNumber=0  TunabilityNumber=1  MinValue=[]  MaxValue=[]  UseSameName=on  MaskValue=upmixer.mix.frw
  TuneTOP4 : TuneVar/TuneTOP  TriggerInit=[1050 707 1220 763]  TopName=flw_mix  TuneName=flw_mix  DataType=single  PackageName=mode  BankNumber=0  TunabilityNumber=1  MinValue=[]  MaxValue=[]  UseSameName=on  MaskValue=upmixer.mix.flw
  TuneTOP5 : TuneVar/TuneTOP  TriggerInit=[1050 572 1220 628]  TopName=gr_mix  TuneName=gr_mix  DataType=single  PackageName=mode  BankNumber=0  TunabilityNumber=1  MinValue=[]  MaxValue=[]  UseSameName=on  MaskValue=upmixer.mix.gl
  TuneTOP6 : TuneVar/TuneTOP  TriggerInit=[1050 437 1220 493]  TopName=gl_mix  TuneName=gl_mix  DataType=single  PackageName=mode  BankNumber=0  TunabilityNumber=1  MinValue=[]  MaxValue=[]  UseSameName=on  MaskValue=upmixer.mix.gl
  MixGains_Front : Outport  VectorParamsAs1DForOutWhenUnconnected=off
  wires:
  TuneTOP6/1 -> Bus Creator/4  "gl"
  TuneTOP5/1 -> Bus Creator/5  "gr"
  TuneTOP4/1 -> Bus Creator/6  "flw"
  TuneTOP3/1 -> Bus Creator/7  "frw"
  TuneTOP2/1 -> Bus Creator/3  "fr"
  TuneTOP1/1 -> Bus Creator/2  "fl"
  TuneTOP/1 -> Bus Creator/1  "dc"
  Bus Creator/1 -> MixGains_Front/1

== system UpmixerLib/Upmixer/mixGains_passenger1 ==
  Bus Creator : BusCreator  Inputs=12
  TuneTOP : TuneVar/TuneTOP  TriggerInit=[1490 612 1660 668]  TopName=LCI1_mix  TuneName=LCI1_mix  DataType=single  PackageName=mode  BankNumber=0  TunabilityNumber=1  MinValue=[]  MaxValue=[]  UseSameName=on  MaskValue=upmixer.mix.LCI1
  TuneTOP1 : TuneVar/TuneTOP  TriggerInit=[1490 712 1660 768]  TopName=LCT1_mix  TuneName=LCT1_mix  DataType=single  PackageName=mode  BankNumber=0  TunabilityNumber=1  MinValue=[]  MaxValue=[]  UseSameName=on  MaskValue=upmixer.mix.LCT1
  TuneTOP10 : TuneVar/TuneTOP  TriggerInit=[1490 412 1660 468]  TopName=RSI1_mix  TuneName=RSI1_mix  DataType=single  PackageName=mode  BankNumber=0  TunabilityNumber=1  MinValue=[]  MaxValue=[]  UseSameName=on  MaskValue=upmixer.mix.RSI1
  TuneTOP11 : TuneVar/TuneTOP  TriggerInit=[1490 512 1660 568]  TopName=RST1_mix  TuneName=RST1_mix  DataType=single  PackageName=mode  BankNumber=0  TunabilityNumber=1  MinValue=[]  MaxValue=[]  UseSameName=on  MaskValue=upmixer.mix.RST1
  TuneTOP2 : TuneVar/TuneTOP  TriggerInit=[1490 -188 1660 -132]  TopName=LFI1_mix  TuneName=LFI1_mix  DataType=single  PackageName=mode  BankNumber=0  TunabilityNumber=1  MinValue=[]  MaxValue=[]  UseSameName=on  MaskValue=upmixer.mix.LFI1
  TuneTOP3 : TuneVar/TuneTOP  TriggerInit=[1490 -88 1660 -32]  TopName=LFT1_mix  TuneName=LFT1_mix  DataType=single  PackageName=mode  BankNumber=0  TunabilityNumber=1  MinValue=[]  MaxValue=[]  UseSameName=on  MaskValue=upmixer.mix.LFT1
  TuneTOP4 : TuneVar/TuneTOP  TriggerInit=[1490 212 1660 268]  TopName=LSI1_mix  TuneName=LSI1_mix  DataType=single  PackageName=mode  BankNumber=0  TunabilityNumber=1  MinValue=[]  MaxValue=[]  UseSameName=on  MaskValue=upmixer.mix.LSI1
  TuneTOP5 : TuneVar/TuneTOP  TriggerInit=[1490 312 1660 368]  TopName=LST1_mix  TuneName=LST1_mix  DataType=single  PackageName=mode  BankNumber=0  TunabilityNumber=1  MinValue=[]  MaxValue=[]  UseSameName=on  MaskValue=upmixer.mix.LST1
  TuneTOP6 : TuneVar/TuneTOP  TriggerInit=[1490 812 1660 868]  TopName=RCI1_mix  TuneName=RCI1_mix  DataType=single  PackageName=mode  BankNumber=0  TunabilityNumber=1  MinValue=[]  MaxValue=[]  UseSameName=on  MaskValue=upmixer.mix.RCI1
  TuneTOP7 : TuneVar/TuneTOP  TriggerInit=[1490 912 1660 968]  TopName=RCT1_mix  TuneName=RCT1_mix  DataType=single  PackageName=mode  BankNumber=0  TunabilityNumber=1  MinValue=[]  MaxValue=[]  UseSameName=on  MaskValue=upmixer.mix.RCT1
  TuneTOP8 : TuneVar/TuneTOP  TriggerInit=[1490 12 1660 68]  TopName=RFI1_mix  TuneName=RFI1_mix  DataType=single  PackageName=mode  BankNumber=0  TunabilityNumber=1  MinValue=[]  MaxValue=[]  UseSameName=on  MaskValue=upmixer.mix.RFI1
  TuneTOP9 : TuneVar/TuneTOP  TriggerInit=[1490 112 1660 168]  TopName=RFT1_mix  TuneName=RFT1_mix  DataType=single  PackageName=mode  BankNumber=0  TunabilityNumber=1  MinValue=[]  MaxValue=[]  UseSameName=on  MaskValue=upmixer.mix.RFT1
  MixGains_Passenger : Outport  VectorParamsAs1DForOutWhenUnconnected=off
  wires:
  TuneTOP11/1 -> Bus Creator/8  "RST1"
  TuneTOP10/1 -> Bus Creator/7  "RSI1"
  TuneTOP9/1 -> Bus Creator/4  "RFT1"
  TuneTOP8/1 -> Bus Creator/3  "RFI1"
  TuneTOP7/1 -> Bus Creator/12  "RCT1"
  TuneTOP6/1 -> Bus Creator/11  "RCI1"
  TuneTOP5/1 -> Bus Creator/6  "LST1"
  TuneTOP4/1 -> Bus Creator/5  "LSI1"
  TuneTOP3/1 -> Bus Creator/2  "LFT1"
  TuneTOP2/1 -> Bus Creator/1  "LFI1"
  TuneTOP1/1 -> Bus Creator/10  "LCT1"
  TuneTOP/1 -> Bus Creator/9  "LCI1"
  Bus Creator/1 -> MixGains_Passenger/1

== system UpmixerLib/Upmixer/conditionallyAddCh2/If Action Subsystem ==
  In1 : Inport
  In2 : Inport  Port=2
  Action Port : ActionPort  ActionPortLabel=else { }
  Out1 : Outport  VectorParamsAs1DForOutWhenUnconnected=off
  Out2 : Outport  Port=2  VectorParamsAs1DForOutWhenUnconnected=off
  wires:
  In1/1 -> Out1/1
  In2/1 -> Out2/1

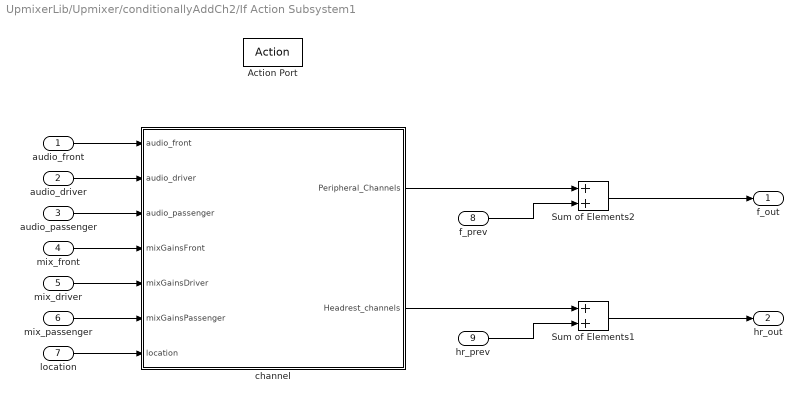
== system UpmixerLib/Upmixer/conditionallyAddCh2/If Action Subsystem1 ==
  audio_front : Inport
  audio_driver : Inport  Port=2
  audio_passenger : Inport  Port=3
  mix_front : Inport  Port=4
  mix_driver : Inport  Port=5
  mix_passenger : Inport  Port=6
  location : Inport  Port=7
  f_prev : Inport  Port=8
  hr_prev : Inport  Port=9
  Action Port : ActionPort  ActionPortLabel=if { }
  Sum of Elements1 : Sum  CollapseMode=Specified dimension  CollapseDim=2
  Sum of Elements2 : Sum  CollapseMode=Specified dimension  CollapseDim=2
  channel : Subsystem
  f_out : Outport  VectorParamsAs1DForOutWhenUnconnected=off
  hr_out : Outport  Port=2  VectorParamsAs1DForOutWhenUnconnected=off
  wires:
  audio_front/1 -> channel/1(audio_front)
  mix_front/1 -> channel/4(mixGainsFront)
  mix_driver/1 -> channel/5(mixGainsDriver)
  mix_passenger/1 -> channel/6(mixGainsPassenger)
  channel/1(Peripheral_Channels) -> Sum of Elements2/1
  f_prev/1 -> Sum of Elements2/2
  Sum of Elements2/1 -> f_out/1
  location/1 -> channel/7(location)
  audio_driver/1 -> channel/2(audio_driver)
  audio_passenger/1 -> channel/3(audio_passenger)
  channel/2(Headrest_channels) -> Sum of Elements1/1
  hr_prev/1 -> Sum of Elements1/2
  Sum of Elements1/1 -> hr_out/1

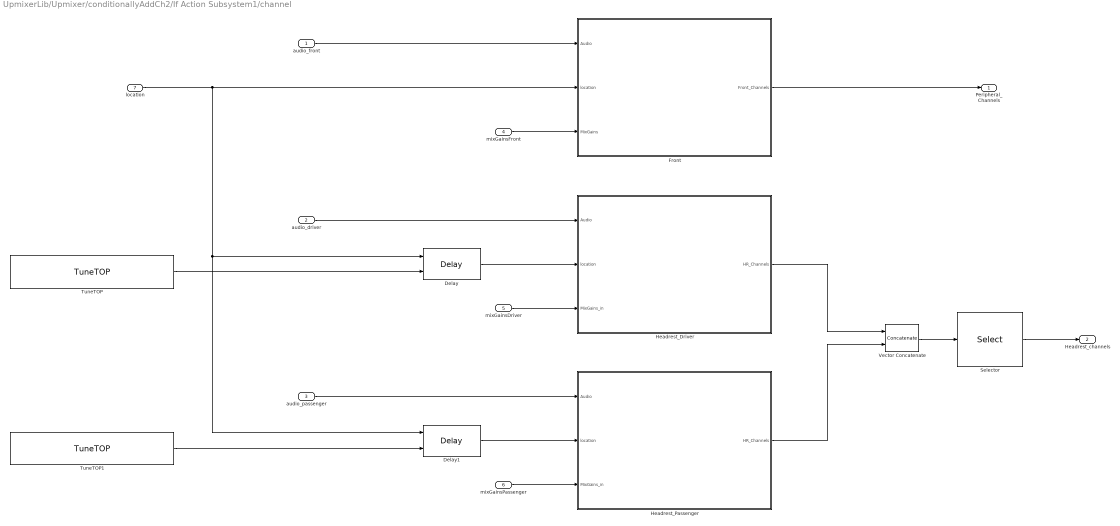
== system UpmixerLib/Upmixer/conditionallyAddCh2/If Action Subsystem1/channel ==
  audio_front : Inport
  audio_driver : Inport  Port=2
  audio_passenger : Inport  Port=3
  mixGainsFront : Inport  Port=4
  mixGainsDriver : Inport  Port=5
  mixGainsPassenger : Inport  Port=6
  location : Inport  Port=7
  Delay : $bdroot/Upmixer/conditionallyAddCh2/If Action Subsystem1/channel/Front/Delay  SystemSampleTime=-1  VariantActivationTime=update diagram  Latency=0  AutoFrameSizeCalculation=off
  Delay1 : $bdroot/Upmixer/conditionallyAddCh2/If Action Subsystem1/channel/Front/Delay  SystemSampleTime=-1  VariantActivationTime=update diagram  Latency=0  AutoFrameSizeCalculation=off
  Front : Subsystem
  Headrest_Driver : Subsystem
  Headrest_Passenger : Subsystem
  Selector : Selector  NumberOfDimensions=2  InputPortWidth=3  IndexOptions=Select all,Index vector (dialog)  Indices=[1 3],[1:(12*upmixer.headrest_count)]  OutputSizes=1,1
  TuneTOP : TuneVar/TuneTOP  TriggerInit=[-530 564 -215 626]  TopName=driver_delay  TuneName=driver_delay  DataType=single  PackageName=mode  BankNumber=0  TunabilityNumber=1  MinValue=[]  MaxValue=[]  UseSameName=on  MaskValue=upmixer.eqdelays.driver
  TuneTOP1 : TuneVar/TuneTOP  TriggerInit=[-530 904 -215 966]  TopName=passenger_delay  TuneName=passenger_delay  DataType=single  PackageName=mode  BankNumber=0  TunabilityNumber=1  MinValue=[]  MaxValue=[]  UseSameName=on  MaskValue=upmixer.eqdelays.passenger
  Vector Concatenate : Concatenate  Mode=Multidimensional array  ConcatenateDimension=2
  Peripheral_Channels : Outport
  Headrest_channels : Outport  Port=2  VectorParamsAs1DForOutWhenUnconnected=off
  wires:
  mixGainsDriver/1 -> Headrest_Driver/3(MixGains_in)
  mixGainsPassenger/1 -> Headrest_Passenger/3(MixGains_in)
  mixGainsFront/1 -> Front/3(MixGains)
  Selector/1 -> Headrest_channels/1
  Vector Concatenate/1 -> Selector/1
  Front/1(Front_Channels) -> Peripheral_Channels/1
  audio_front/1 -> Front/1(Audio)
  audio_driver/1 -> Headrest_Driver/1(Audio)
  audio_passenger/1 -> Headrest_Passenger/1(Audio)
  Headrest_Driver/1(HR_Channels) -> Vector Concatenate/1
  Headrest_Passenger/1(HR_Channels) -> Vector Concatenate/2
  location/1 -> Delay1/1, Delay/1, Front/2(location)
  TuneTOP/1 -> Delay/2
  Delay/1 -> Headrest_Driver/2(location)
  Delay1/1 -> Headrest_Passenger/2(location)
  TuneTOP1/1 -> Delay1/2

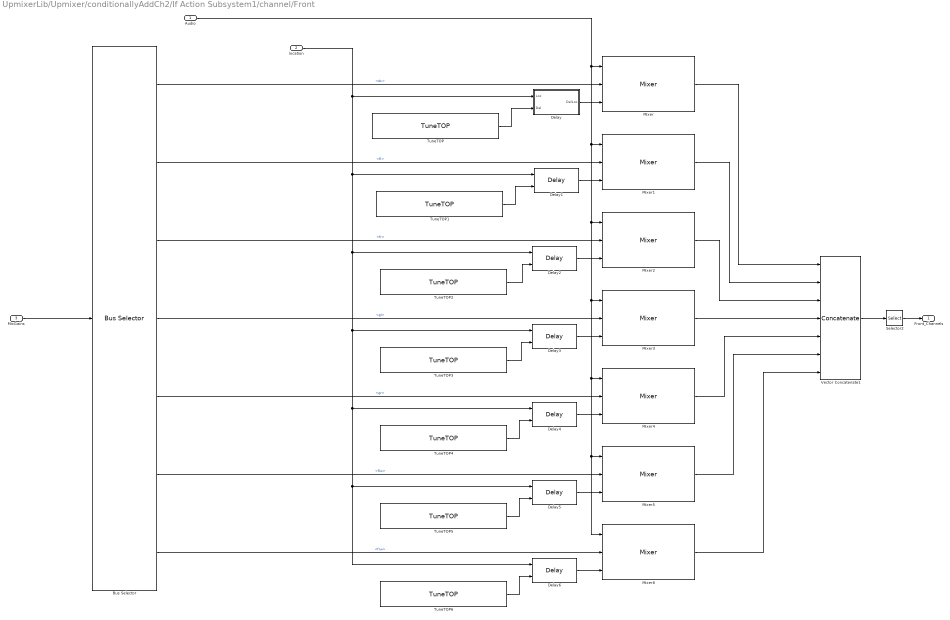
== system UpmixerLib/Upmixer/conditionallyAddCh2/If Action Subsystem1/channel/Front ==
  Audio : Inport
  location : Inport  Port=2
  MixGains : Inport  Port=3
  Bus Selector : BusSelector  OutputSignals=dc,fl,fr,gl,gr,flw,frw
  Delay : Subsystem  TreatAsAtomicUnit=on
  Delay{1..6} (6 alike) : $bdroot/Upmixer/conditionallyAddCh2/If Action Subsystem1/channel/Front/Delay  SystemSampleTime=-1  VariantActivationTime=update diagram  Latency=0  AutoFrameSizeCalculation=off
  Mixer{,1..6} (7 alike) : MixerLib/Mixer  SystemSampleTime=-1  VariantActivationTime=update diagram  Latency=0  AutoFrameSizeCalculation=off
  Selector2 : Selector  NumberOfDimensions=2  InputPortWidth=3  IndexOptions=Select all,Index vector (dialog)  Indices=[1 32],[1:upmixer.front_peripheral_channel_count]  OutputSizes=1,1
  TuneTOP : TuneVar/TuneTOP  TriggerInit=[700 229 1015 291]  TopName=dc_delay  TuneName=dc_delay  DataType=single  PackageName=mode  BankNumber=0  TunabilityNumber=1  MinValue=[]  MaxValue=[]  UseSameName=on  MaskValue=upmixer.eqdelays.dc
  TuneTOP1 : TuneVar/TuneTOP  TriggerInit=[710 424 1025 486]  TopName=fl_delay  TuneName=fl_delay  DataType=single  PackageName=mode  BankNumber=0  TunabilityNumber=1  MinValue=[]  MaxValue=[]  UseSameName=on  MaskValue=upmixer.eqdelays.fl
  TuneTOP2 : TuneVar/TuneTOP  TriggerInit=[720 619 1035 681]  TopName=fr_delay  TuneName=fr_delay  DataType=single  PackageName=mode  BankNumber=0  TunabilityNumber=1  MinValue=[]  MaxValue=[]  UseSameName=on  MaskValue=upmixer.eqdelays.fr
  TuneTOP3 : TuneVar/TuneTOP  TriggerInit=[720 814 1035 876]  TopName=gl_delay  TuneName=gl_delay  DataType=single  PackageName=mode  BankNumber=0  TunabilityNumber=1  MinValue=[]  MaxValue=[]  UseSameName=on  MaskValue=upmixer.eqdelays.gl
  TuneTOP4 : TuneVar/TuneTOP  TriggerInit=[720 1009 1035 1071]  TopName=gr_delay  TuneName=gr_delay  DataType=single  PackageName=mode  BankNumber=0  TunabilityNumber=1  MinValue=[]  MaxValue=[]  UseSameName=on  MaskValue=upmixer.eqdelays.gr
  TuneTOP5 : TuneVar/TuneTOP  TriggerInit=[720 1204 1035 1266]  TopName=flw_delay  TuneName=flw_delay  DataType=single  PackageName=mode  BankNumber=0  TunabilityNumber=1  MinValue=[]  MaxValue=[]  UseSameName=on  MaskValue=upmixer.eqdelays.flw
  TuneTOP6 : TuneVar/TuneTOP  TriggerInit=[720 1399 1035 1461]  TopName=frw_delay  TuneName=frw_delay  DataType=single  PackageName=mode  BankNumber=0  TunabilityNumber=1  MinValue=[]  MaxValue=[]  UseSameName=on  MaskValue=upmixer.eqdelays.frw
  Vector Concatenate1 : Concatenate  NumInputs=7  Mode=Multidimensional array  ConcatenateDimension=2
  Front_Channels : Outport  VectorParamsAs1DForOutWhenUnconnected=off
  wires:
  MixGains/1 -> Bus Selector/1
  Selector2/1 -> Front_Channels/1
  Vector Concatenate1/1 -> Selector2/1
  Bus Selector/7 -> Mixer6/2  "<frw>"
  Bus Selector/6 -> Mixer5/2  "<flw>"
  Bus Selector/5 -> Mixer4/2  "<gr>"
  Bus Selector/4 -> Mixer3/2  "<gl>"
  Bus Selector/3 -> Mixer2/2  "<fr>"
  Mixer6/1 -> Vector Concatenate1/7
  Mixer5/1 -> Vector Concatenate1/6
  Mixer4/1 -> Vector Concatenate1/5
  Mixer3/1 -> Vector Concatenate1/4
  Mixer2/1 -> Vector Concatenate1/3
  Mixer/1 -> Vector Concatenate1/1
  Audio/1 -> Mixer6/1, Mixer5/1, Mixer4/1, Mixer3/1, Mixer2/1, Mixer1/1, Mixer/1
  Mixer1/1 -> Vector Concatenate1/2
  Bus Selector/2 -> Mixer1/2  "<fl>"
  Bus Selector/1 -> Mixer/2  "<dc>"
  location/1 -> Delay/1(Loc), Delay1/1, Delay2/1, Delay3/1, Delay4/1, Delay6/1, Delay5/1
  TuneTOP1/1 -> Delay1/2
  Delay1/1 -> Mixer1/3
  TuneTOP2/1 -> Delay2/2
  Delay2/1 -> Mixer2/3
  TuneTOP3/1 -> Delay3/2
  Delay3/1 -> Mixer3/3
  TuneTOP4/1 -> Delay4/2
  Delay4/1 -> Mixer4/3
  TuneTOP5/1 -> Delay5/2
  Delay5/1 -> Mixer5/3
  TuneTOP6/1 -> Delay6/2
  Delay6/1 -> Mixer6/3
  TuneTOP/1 -> Delay/2(Del)
  Delay/1(DelLoc) -> Mixer/3

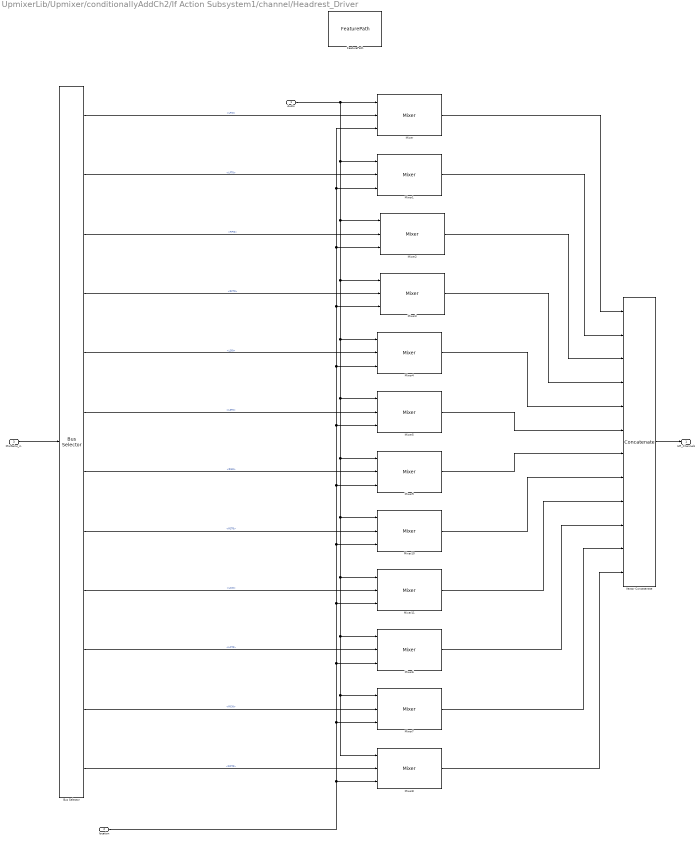
== system UpmixerLib/Upmixer/conditionallyAddCh2/If Action Subsystem1/channel/Headrest_Driver ==
  Audio : Inport
  location : Inport  Port=2
  MixGains_in : Inport  Port=3
  Bus Selector : BusSelector  OutputSignals=LFI0,LFT0,RFI0,RFT0,LSI0,LST0,RSI0,RST0,LCI0,LCT0,RCI0,RCT0
  FeaturePath : FeaturePath/FeaturePath  FeatureName=Driver_  IsGroup=off  GroupNumber=-1  DeclarePackages=off  PackageNames=mode,carModel  IsToolGroup=off  TriggerInit=[30 284 210 401]
  Mixer{,1..11} (12 alike) : MixerLib/Mixer  SystemSampleTime=-1  VariantActivationTime=update diagram  Latency=0  AutoFrameSizeCalculation=off
  Vector Concatenate : Concatenate  NumInputs=12  Mode=Multidimensional array  ConcatenateDimension=2
  HR_Channels : Outport  VectorParamsAs1DForOutWhenUnconnected=off
  wires:
  location/1 -> Mixer/3, Mixer1/3, Mixer2/3, Mixer3/3, Mixer4/3, Mixer5/3, Mixer9/3, Mixer10/3, Mixer11/3, Mixer6/3, Mixer7/3, Mixer8/3
  MixGains_in/1 -> Bus Selector/1
  Vector Concatenate/1 -> HR_Channels/1
  Audio/1 -> Mixer8/1, Mixer7/1, Mixer6/1, Mixer11/1, Mixer10/1, Mixer9/1, Mixer5/1, Mixer4/1, Mixer3/1, Mixer2/1, Mixer1/1, Mixer/1
  Bus Selector/11 -> Mixer7/2  "<RCI0>"
  Bus Selector/7 -> Mixer9/2  "<RSI0>"
  Bus Selector/9 -> Mixer11/2  "<LCI0>"
  Bus Selector/8 -> Mixer10/2  "<RST0>"
  Bus Selector/10 -> Mixer6/2  "<LCT0>"
  Mixer10/1 -> Vector Concatenate/8
  Mixer6/1 -> Vector Concatenate/10
  Mixer9/1 -> Vector Concatenate/7
  Mixer11/1 -> Vector Concatenate/9
  Mixer8/1 -> Vector Concatenate/12
  Mixer7/1 -> Vector Concatenate/11
  Bus Selector/12 -> Mixer8/2  "<RCT0>"
  Bus Selector/6 -> Mixer5/2  "<LST0>"
  Mixer4/1 -> Vector Concatenate/5
  Mixer1/1 -> Vector Concatenate/2
  Bus Selector/5 -> Mixer4/2  "<LSI0>"
  Bus Selector/2 -> Mixer1/2  "<LFT0>"
  Bus Selector/1 -> Mixer/2  "<LFI0>"
  Bus Selector/4 -> Mixer3/2  "<RFT0>"
  Mixer/1 -> Vector Concatenate/1
  Bus Selector/3 -> Mixer2/2  "<RFI0>"
  Mixer2/1 -> Vector Concatenate/3
  Mixer5/1 -> Vector Concatenate/6
  Mixer3/1 -> Vector Concatenate/4

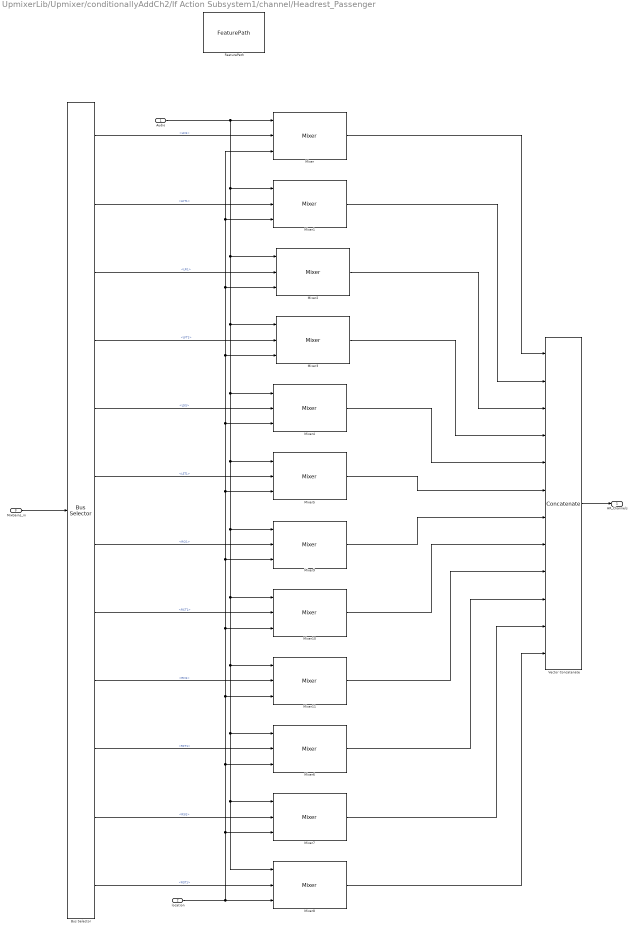
== system UpmixerLib/Upmixer/conditionallyAddCh2/If Action Subsystem1/channel/Headrest_Passenger ==
  Audio : Inport
  location : Inport  Port=2
  MixGains_in : Inport  Port=3
  Bus Selector : BusSelector  OutputSignals=LCI1,LCT1,LFI1,LFT1,LSI1,LST1,RCI1,RCT1,RFI1,RFT1,RSI1,RST1
  FeaturePath : FeaturePath/FeaturePath  FeatureName=Passenger_  IsGroup=off  GroupNumber=-1  DeclarePackages=off  PackageNames=mode,carModel  IsToolGroup=off  TriggerInit=[30 284 210 401]
  Mixer{,1..11} (12 alike) : MixerLib/Mixer  SystemSampleTime=-1  VariantActivationTime=update diagram  Latency=0  AutoFrameSizeCalculation=off
  Vector Concatenate : Concatenate  NumInputs=12  Mode=Multidimensional array  ConcatenateDimension=2
  HR_Channels : Outport  VectorParamsAs1DForOutWhenUnconnected=off
  wires:
  Mixer3/1 -> Vector Concatenate/4
  Mixer5/1 -> Vector Concatenate/6
  Mixer2/1 -> Vector Concatenate/3
  Bus Selector/3 -> Mixer2/2  "<LFI1>"
  Mixer/1 -> Vector Concatenate/1
  Bus Selector/4 -> Mixer3/2  "<LFT1>"
  Bus Selector/1 -> Mixer/2  "<LCI1>"
  Bus Selector/2 -> Mixer1/2  "<LCT1>"
  Bus Selector/5 -> Mixer4/2  "<LSI1>"
  Mixer1/1 -> Vector Concatenate/2
  Mixer4/1 -> Vector Concatenate/5
  Bus Selector/6 -> Mixer5/2  "<LST1>"
  Bus Selector/12 -> Mixer8/2  "<RST1>"
  Mixer7/1 -> Vector Concatenate/11
  Mixer8/1 -> Vector Concatenate/12
  Mixer11/1 -> Vector Concatenate/9
  Mixer9/1 -> Vector Concatenate/7
  Mixer6/1 -> Vector Concatenate/10
  Mixer10/1 -> Vector Concatenate/8
  Bus Selector/10 -> Mixer6/2  "<RFT1>"
  Bus Selector/8 -> Mixer10/2  "<RCT1>"
  Bus Selector/9 -> Mixer11/2  "<RFI1>"
  Bus Selector/7 -> Mixer9/2  "<RCI1>"
  Bus Selector/11 -> Mixer7/2  "<RSI1>"
  Audio/1 -> Mixer5/1, Mixer10/1, Mixer8/1, Mixer7/1, Mixer6/1, Mixer11/1, Mixer9/1, Mixer4/1, Mixer3/1, Mixer2/1, Mixer1/1, Mixer/1
  Vector Concatenate/1 -> HR_Channels/1
  MixGains_in/1 -> Bus Selector/1
  location/1 -> Mixer10/3, Mixer9/3, Mixer/3, Mixer1/3, Mixer2/3, Mixer3/3, Mixer4/3, Mixer5/3, Mixer11/3, Mixer6/3, Mixer7/3, Mixer8/3

== system UpmixerLib/Upmixer/conditionallyAddCh2/If Action Subsystem1/channel/Front/Delay ==
  Loc : Inport
  Del : Inport  Port=2
  Delay : Delay  DelayLengthSource=Input port  DelayLengthUpperLimit=3  InputProcessing=Columns as channels (frame based)
      settings: InputPortMap=u0,p1
  DelLoc : Outport
  wires:
  Del/1 -> Delay/2
  Delay/1 -> DelLoc/1
  Loc/1 -> Delay/1
